simulink model "roll_dynamics_controller_simulink"  (R2023a)
settings: Solver=VariableStepAuto  StartTime=0.0  StopTime=8  RelTol=1e-3
settings Model: ExtModeTrigDuration=100  Creator=Shen Zeng  LastModifiedBy=prince
settings SolverCC: AlgebraicLoopSolver=TrustRegion
settings DataIOCC: SaveOutput=off  ReturnWorkspaceOutputs=off  StateSaveName=tmp_raccel_xout  SignalLoggingName=tmp_raccel_logsout
settings OptimizationCC: EfficientMapNaN2IntZero=off
settings DebuggingCC: UnconnectedInputMsg=warning  UnconnectedOutputMsg=warning  UnconnectedLineMsg=warning  ArithmeticOperatorsInVariantConditions=warning
settings HardwareCC: TargetBitPerLong=64  TargetBitPerPointer=64  TargetBitPerSizeT=64  TargetBitPerPtrDiffT=64  TargetLongLongMode=on  TargetIntDivRoundTo=Zero  TargetEndianess=LittleEndian  TargetWordSize=64  TargetHWDeviceType=MATLAB Host  ProdEqTarget=off
settings ModelReferenceCC: EnableRefExpFcnMdlSchedulingChecks=on
settings SFSimCC: SimUseLocalCustomCode=off  CustomCodeUndefinedFunction=UseInterfaceOnly
settings RTWCC: SystemTargetFile=raccel.tlc  TemplateMakefile=raccel_default_tmf  RTWVerbose=off  RTWUseLocalCustomCode=off  RTWUseSimCustomCode=on
settings CodeAppCC: GenerateComments=off  MaxIdLength=128  SimulinkBlockComments=off
settings RaccelTargetCC: OptimizeReductions=off  ENABLE_SLEXEC_SSBRIDGE=0  RTWCAPISignals=off  RTWCAPIParams=on  RTWCAPIRootIO=off

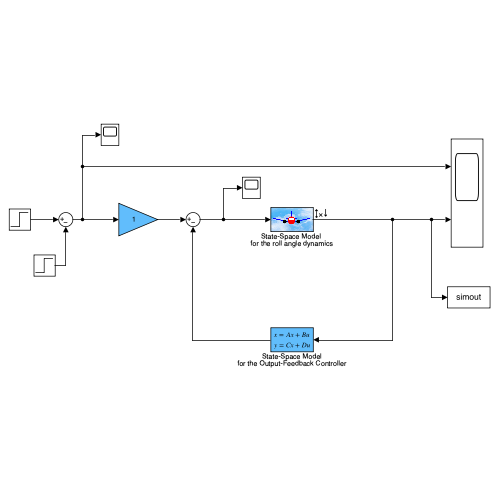
[thumbnail: Simulink's stored preview of the top-level diagram]
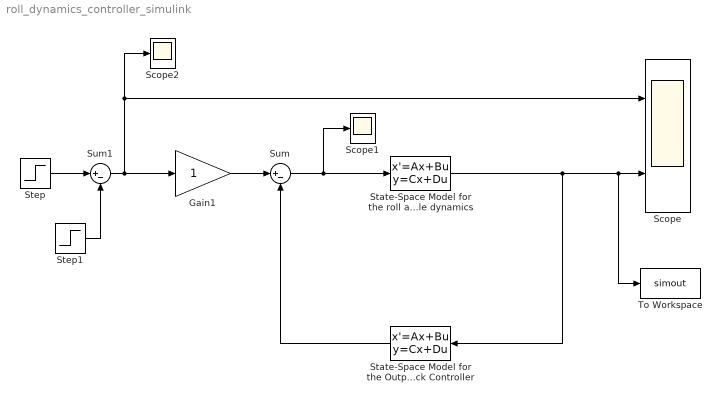
== system roll_dynamics_controller_simulink ==
  Gain1 : Gain
  Scope : Scope  NumInputPorts=2
  Scope1 : Scope
  Scope2 : Scope
  "State-Space Model for the Output-Feedback Controller " : StateSpace  A=[0 1; 0 0]  B=[0;1]  C=[0 0]  D=2  InitialCondition=[0 ; 0]
  State-Space Model for the roll angle dynamics : StateSpace  A=[0 1 ; 0 0]  B=[0;1]  C=[1 , 0 ]  D=0  InitialCondition=[0 ; 0]
      mask Display: image('airplane_icon.png');
  Step : Step  After=deg2rad(30)  SampleTime=0
  Step1 : Step  Time=5  After=deg2rad(30)  SampleTime=0
  Sum : Sum  Inputs=|+-
  Sum1 : Sum  Inputs=|+-
  To Workspace : ToWorkspace  VariableName=simout  SaveFormat=Timeseries  SampleTime=0.05
  wires:
  Sum/1 -> Scope1/1, State-Space Model for the roll angle dynamics/1
  Gain1/1 -> Sum/1
  State-Space Model for the roll angle dynamics/1 -> To Workspace/1, Scope/2, "State-Space Model for the Output-Feedback Controller "/1
  Step/1 -> Sum1/1
  Step1/1 -> Sum1/2
  Sum1/1 -> Scope2/1, Scope/1, Gain1/1
  "State-Space Model for the Output-Feedback Controller "/1 -> Sum/2
